simulink model "HW2b"  (Simulink 8.5)
settings: Solver=ode45  StartTime=0.0  StopTime=1000  MaxStep=0.1  MinStep=0.0001  RelTol=1e-3  AbsTol=1e-3
settings Model: Creator=Hybrid Pederson  LastModifiedBy=ccpc50
settings DataIOCC: SaveOutput=off  SaveTime=off
settings OptimizationCC: InitFltsAndDblsToZero=on
settings DebuggingCC: SaveWithParameterizedLinksMsg=none  SolverPrmCheckMsg=warning  FcnCallInpInsideContextMsg=UseLocalSettings
settings GRTTargetCC: TargetFcnLib=ansi_tfl_tmw.mat

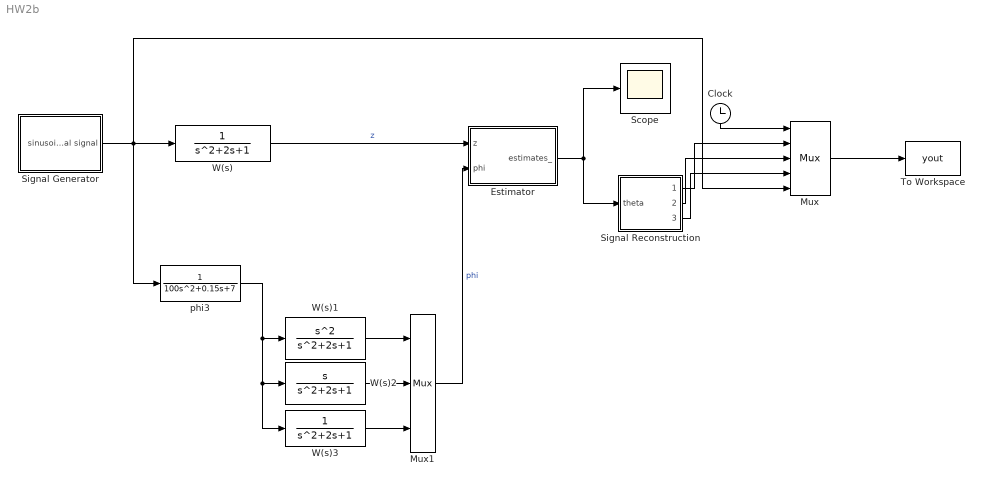
== system HW2b ==
  Clock : Clock
  Estimator : Subsystem
      mask Display: disp('Parameter\nEstimation')
  Mux : Mux  Inputs=5
  Mux1 : Mux  Inputs=3
  Scope : Scope
      settings: TimeRange=50  YMin=-20.000000  YMax=20.000000
  Signal Generator : Subsystem
      mask Display: plot(sin([0.0:0.1:6.3])
  Signal Reconstruction : Subsystem
      mask Display: plot(sin([0.0:0.1:6.3]))
  To Workspace : ToWorkspace  VariableName=yout
      settings: MaxDataPoints=5000
  W(s) : TransferFcn
  W(s)1 : TransferFcn  Numerator=[1 0 0]
  W(s)2 : TransferFcn  Numerator=[1 0]
  W(s)3 : TransferFcn
  phi3 : TransferFcn  Denominator=[100 0.15 7]
  wires:
  Signal Reconstruction/2(est_phase) -> Mux/3
  Mux/1 -> To Workspace/1
  Clock/1 -> Mux/1
  Estimator/1(estimates_) -> Signal Reconstruction/1(theta), Scope/1
  Signal Reconstruction/3(est_signal) -> Mux/4
  Signal Reconstruction/1(est_mag) -> Mux/2
  Signal Generator/1(sinusoidal signal) -> W(s)/1, Mux/5, phi3/1
  Mux1/1 -> Estimator/2(phi)  "phi"
  phi3/1 -> W(s)1/1, W(s)3/1, W(s)2/1
  W(s)/1 -> Estimator/1(z)  "z"
  W(s)1/1 -> Mux1/1
  W(s)2/1 -> Mux1/2
  W(s)3/1 -> Mux1/3

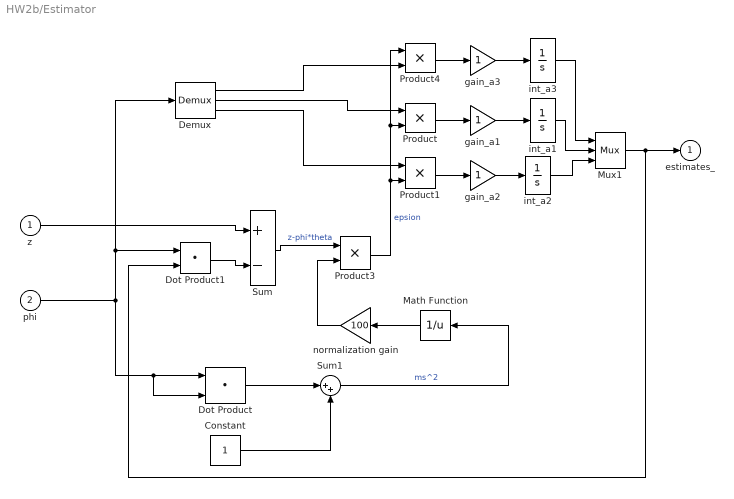
== system HW2b/Estimator ==
  z : Inport
  phi : Inport  Port=2
  Constant : Constant
  Demux : Demux  Outputs=3
  Dot Product : DotProduct  InputSameDT=on  OutDataTypeStr=Inherit: Inherit via internal rule
  Dot Product1 : DotProduct  InputSameDT=on  OutDataTypeStr=Inherit: Inherit via internal rule
  Math Function : Math  Operator=reciprocal  SaturateOnIntegerOverflow=on
  Mux1 : Mux  Inputs=3
  Product{,1,3..4} (4 alike) : Product  SaturateOnIntegerOverflow=on  RndMeth=Zero  InputSameDT=on  OutDataTypeStr=Inherit: Same as first input
  Sum : Sum  Inputs=+-  SaturateOnIntegerOverflow=on  InputSameDT=on  OutDataTypeStr=Inherit: Same as first input
  Sum1 : Sum  Inputs=|++
  gain_a1 : Gain  SaturateOnIntegerOverflow=on  OutDataTypeStr=Inherit: Same as input  ParamDataTypeStr=Inherit: Same as input
  gain_a2 : Gain  SaturateOnIntegerOverflow=on  OutDataTypeStr=Inherit: Same as input  ParamDataTypeStr=Inherit: Same as input
  gain_a3 : Gain  SaturateOnIntegerOverflow=on  OutDataTypeStr=Inherit: Same as input  ParamDataTypeStr=Inherit: Same as input
  int_a1 : Integrator
  int_a2 : Integrator
  int_a3 : Integrator
  normalization gain : Gain  Gain=100  SaturateOnIntegerOverflow=on  OutDataTypeStr=Inherit: Same as input  ParamDataTypeStr=Inherit: Same as input
  estimates_ : Outport
  wires:
  z/1 -> Sum/1
  normalization gain/1 -> Product3/2
  Mux1/1 -> Dot Product1/2, estimates_/1
  Math Function/1 -> normalization gain/1
  Product1/1 -> gain_a2/1
  gain_a2/1 -> int_a2/1
  Product/1 -> gain_a1/1
  gain_a1/1 -> int_a1/1
  Dot Product1/1 -> Sum/2
  Product3/1 -> Product4/1, Product/2, Product1/2  "epsion"
  Sum/1 -> Product3/1  "z-phi*theta"
  phi/1 -> Demux/1, Dot Product1/1, Dot Product/2, Dot Product/1
  gain_a3/1 -> int_a3/1
  Product4/1 -> gain_a3/1
  Demux/1 -> Product4/2
  Demux/2 -> Product/1
  Demux/3 -> Product1/1
  Dot Product/1 -> Sum1/1
  Constant/1 -> Sum1/2
  Sum1/1 -> Math Function/1  "ms^2"
  int_a3/1 -> Mux1/1
  int_a1/1 -> Mux1/2
  int_a2/1 -> Mux1/3

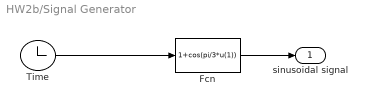
== system HW2b/Signal Generator ==
  Fcn : Fcn  Expr=1+cos(pi/3*u(1))
      mask Display: disp('A sin(wt+p)')
  Time : Clock
  sinusoidal signal : Outport
  wires:
  Time/1 -> Fcn/1
  Fcn/1 -> sinusoidal signal/1

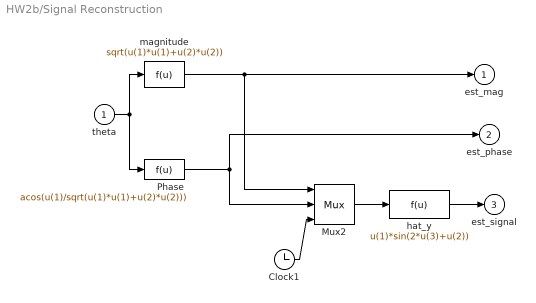
== system HW2b/Signal Reconstruction ==
  theta : Inport
  Clock1 : Clock
  Mux2 : Mux  Inputs=3
  Phase : Fcn  Expr=acos(u(1)/sqrt(u(1)*u(1)+u(2)*u(2)))
      mask Display: disp('P')
  hat_y : Fcn  Expr=u(1)*sin(2*u(3)+u(2))
      mask Display: disp('Asin(wt+p)')
  magnitude : Fcn  Expr=sqrt(u(1)*u(1)+u(2)*u(2))
      mask Display: disp('A')
  est_mag : Outport
  est_phase : Outport  Port=2
  est_signal : Outport  Port=3
  wires:
  Mux2/1 -> hat_y/1
  Clock1/1 -> Mux2/3
  theta/1 -> Phase/1, magnitude/1
  Phase/1 -> Mux2/2, est_phase/1
  magnitude/1 -> Mux2/1, est_mag/1
  hat_y/1 -> est_signal/1
